simulink model "test_matrixmul"  (R2019a)
settings: Solver=VariableStepAuto  StartTime=0.0  StopTime=10.0  RelTol=1e-3
values from neighbouring files (symbols this model uses):
  magic = fread(fp, 1, 'int32', 0)    [loadMNISTImagesTestLE.m]    (also in loadMNISTImagesTrainLE.m)
libraries: ad_blocks x5
settings Model: Creator=eruffaldi  LastModifiedBy=eruffaldi

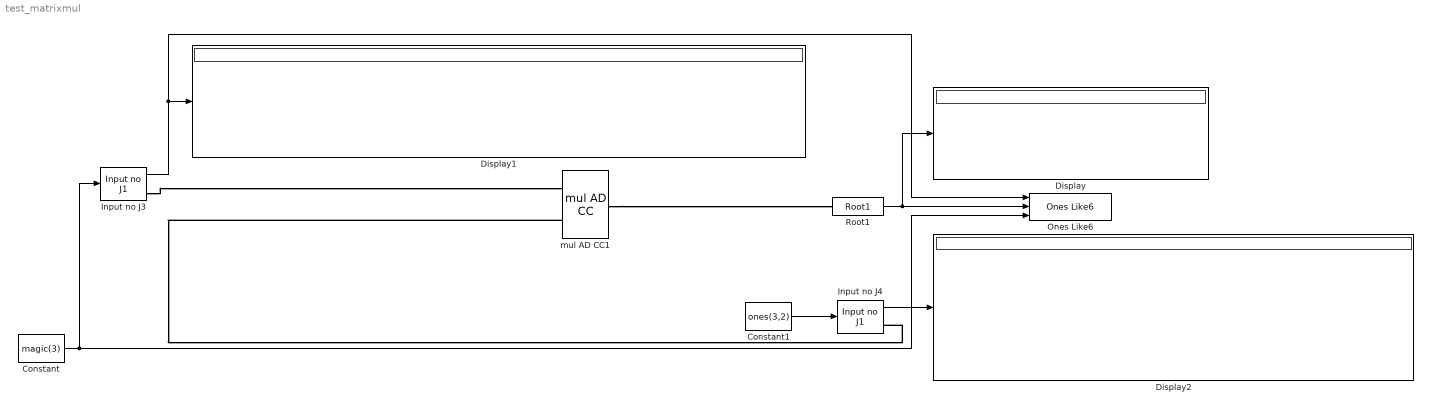
== system test_matrixmul ==
  Constant : Constant  Value=magic(3)
  Constant1 : Constant  Value=ones(3,2)
  Display : Display
  Display1 : Display
  Display2 : Display
  Input no J3 : ad_blocks/Input no J1  SystemSampleTime=-1
  Input no J4 : ad_blocks/Input no J1  SystemSampleTime=-1
  Ones Like6 : ad_blocks/Ones Like6  SimulateUsing=Code generation
  Root1 : ad_blocks/Root1  Description=Top level AD block: gets the incoming value, pushes the multivalued gradient  SystemSampleTime=-1
  mul AD CC1 : ad_blocks/mul AD CC  SystemSampleTime=-1
  wires:
  Constant1/1 -> Input no J4/1
  Root1/1 -> Display/1, Ones Like6/2
  Constant/1 -> Ones Like6/3, Input no J3/1
  Input no J4/1 -> Display2/1
  Input no J3/1 -> Display1/1, Ones Like6/1
  connections:
  mul AD CC1/RConn1 -- Root1/LConn1
  Input no J3/RConn1 -- mul AD CC1/LConn1
  mul AD CC1/LConn2 -- Input no J4/RConn1
